simulink model "SigProcess"  (R2022b)
settings: Solver=FixedStepDiscrete  StartTime=0.0  StopTime=10.0  FixedStep=0.001  RelTol=1e-3
undefined symbols (not defined in the file): cClCddAdc_D_u16ADNum, cClCddAdc_D_u8FilterType, cClCddAdc_D_u8RawValueNum, cTmAfCtrl_Te_s32ShttrPosnColdOnHp
libraries: simulink x132
(part 2 of 7)

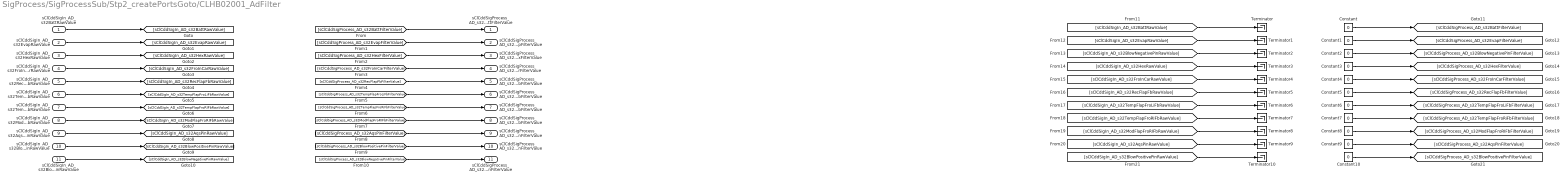
== system SigProcess/SigProcessSub/Stp2_createPortsGoto/CLHB02001_AdFilter ==
  sClCddSigIn_AD_s32BattRawValue : Inport  Description=低压电池AD值  OutDataTypeStr=single
  sClCddSigIn_AD_s32EvapRawValue : Inport  Description=空调箱蒸发器原始AD值  Port=2  OutDataTypeStr=single
  sClCddSigIn_AD_s32HexRawValue : Inport  Description=空调箱热交换器原始AD值  Port=3  OutDataTypeStr=single
  sClCddSigIn_AD_s32FroInCarRawValue : Inport  Description=前排车内温度传感器AD值  Port=4  OutDataTypeStr=single
  sClCddSigIn_AD_s32RecFlapFbRawValue : Inport  Description=内循环风门电机位置反馈  Port=5  OutDataTypeStr=single
  sClCddSigIn_AD_s32TempFlapFroLiFbRawValue : Inport  Description=前左风门电机位置反馈  Port=6  OutDataTypeStr=single
  sClCddSigIn_AD_s32TempFlapFroRIFbRawValue : Inport  Description=前右风门电机位置反馈  Port=7  OutMin=0  OutMax=2048  OutDataTypeStr=single
  sClCddSigIn_AD_s32ModFlapFroRIFbRawValue : Inport  Description=模式风门电机位置反馈  Port=8  OutMin=0  OutMax=2048  OutDataTypeStr=single
  sClCddSigIn_AD_s32AqsPinRawValue : Inport  Description=AQSPWM驱动芯片诊断PIN脚AD值  Port=9  OutMin=0  OutMax=2048  OutDataTypeStr=single
  sClCddSigIn_AD_s32BlowPositivePinRawValue : Inport  Description=鼓风机调速电机正极反馈  Port=10  OutMin=0  OutMax=2048  OutDataTypeStr=single
  sClCddSigIn_AD_s32BlowNegativePinRawValue : Inport  Description=鼓风机调速电机负极反馈  Port=11  OutMin=0  OutMax=2048  OutDataTypeStr=single
  Constant{,1..10} (11 alike) : Constant  Value=0  OutDataTypeStr=single
  Terminator{,1..10} (11 alike) : Terminator
  sClCddSigProcess_AD_s32BattFilterValue : Outport  Description=低压电池滤波后AD值  OutMin=0  OutMax=2048  OutDataTypeStr=single
  sClCddSigProcess_AD_s32EvapFilterValue : Outport  Description=空调箱蒸发器滤波后AD值  Port=2  OutMin=0  OutMax=2048  OutDataTypeStr=single
  sClCddSigProcess_AD_s32HexFilterValue : Outport  Description=空调箱热交换器滤波后AD值  Port=3  OutMin=0  OutMax=2048  OutDataTypeStr=single
  sClCddSigProcess_AD_s32FroInCarFilterValue : Outport  Description=前排车内温度传感器滤波后AD值  Port=4  OutMin=0  OutMax=2048  OutDataTypeStr=single
  sClCddSigProcess_AD_s32RecFlapFbFilterValue : Outport  Description=内循环风门电机位置反馈滤波值  Port=5  OutMin=0  OutMax=2048  OutDataTypeStr=single
  sClCddSigProcess_AD_s32TempFlapFroLiFbFilterValue : Outport  Description=前左风门电机位置反馈滤波值  Port=6  OutMin=0  OutMax=2048  OutDataTypeStr=single
  sClCddSigProcess_AD_s32TempFlapFroRiFbFilterValue : Outport  Description=前右风门电机位置反馈滤波值  Port=7  OutMin=0  OutMax=2048  OutDataTypeStr=single
  sClCddSigProcess_AD_s32ModFlapFroRIFbFilterValue : Outport  Description=模式风门电机位置反馈滤波值  Port=8  OutMin=0  OutMax=2048  OutDataTypeStr=single
  sClCddSigProcess_AD_s32AqsPinFilterValue : Outport  Description=AQSPWM驱动芯片诊断PIN脚滤波值  Port=9  OutMin=0  OutMax=2048  OutDataTypeStr=single
  sClCddSigProcess_AD_s32BlowPositivePinFilterValue : Outport  Description=鼓风机调速电机正极反馈滤波值  Port=10  OutMin=0  OutMax=2048  OutDataTypeStr=single
  sClCddSigProcess_AD_s32BlowNegativePinFilterValue : Outport  Description=鼓风机调速电机负极反馈滤波值  Port=11  OutMin=0  OutMax=2048  OutDataTypeStr=single
  wires:
  sClCddSigIn_AD_s32BattRawValue/1 -> [sClCddSigIn_AD_s32BattRawValue]
  sClCddSigIn_AD_s32EvapRawValue/1 -> [sClCddSigIn_AD_s32EvapRawValue]
  sClCddSigIn_AD_s32HexRawValue/1 -> [sClCddSigIn_AD_s32HexRawValue]
  sClCddSigIn_AD_s32FroInCarRawValue/1 -> [sClCddSigIn_AD_s32FroInCarRawValue]
  sClCddSigIn_AD_s32RecFlapFbRawValue/1 -> [sClCddSigIn_AD_s32RecFlapFbRawValue]
  sClCddSigIn_AD_s32TempFlapFroLiFbRawValue/1 -> [sClCddSigIn_AD_s32TempFlapFroLiFbRawValue]
  sClCddSigIn_AD_s32TempFlapFroRIFbRawValue/1 -> [sClCddSigIn_AD_s32TempFlapFroRIFbRawValue]
  sClCddSigIn_AD_s32ModFlapFroRIFbRawValue/1 -> [sClCddSigIn_AD_s32ModFlapFroRIFbRawValue]
  sClCddSigIn_AD_s32AqsPinRawValue/1 -> [sClCddSigIn_AD_s32AqsPinRawValue]
  sClCddSigIn_AD_s32BlowPositivePinRawValue/1 -> [sClCddSigIn_AD_s32BlowPositivePinRawValue]
  sClCddSigIn_AD_s32BlowNegativePinRawValue/1 -> [sClCddSigIn_AD_s32BlowNegativePinRawValue]
  [sClCddSigProcess_AD_s32BattFilterValue] -> sClCddSigProcess_AD_s32BattFilterValue/1
  [sClCddSigProcess_AD_s32EvapFilterValue] -> sClCddSigProcess_AD_s32EvapFilterValue/1
  [sClCddSigProcess_AD_s32HexFilterValue] -> sClCddSigProcess_AD_s32HexFilterValue/1
  [sClCddSigProcess_AD_s32FroInCarFilterValue] -> sClCddSigProcess_AD_s32FroInCarFilterValue/1
  [sClCddSigProcess_AD_s32RecFlapFbFilterValue] -> sClCddSigProcess_AD_s32RecFlapFbFilterValue/1
  [sClCddSigProcess_AD_s32TempFlapFroLiFbFilterValue] -> sClCddSigProcess_AD_s32TempFlapFroLiFbFilterValue/1
  [sClCddSigProcess_AD_s32TempFlapFroRiFbFilterValue] -> sClCddSigProcess_AD_s32TempFlapFroRiFbFilterValue/1
  [sClCddSigProcess_AD_s32ModFlapFroRIFbFilterValue] -> sClCddSigProcess_AD_s32ModFlapFroRIFbFilterValue/1
  [sClCddSigProcess_AD_s32AqsPinFilterValue] -> sClCddSigProcess_AD_s32AqsPinFilterValue/1
  [sClCddSigProcess_AD_s32BlowPositivePinFilterValue] -> sClCddSigProcess_AD_s32BlowPositivePinFilterValue/1
  [sClCddSigProcess_AD_s32BlowNegativePinFilterValue] -> sClCddSigProcess_AD_s32BlowNegativePinFilterValue/1
  Constant/1 -> [sClCddSigProcess_AD_s32BattFilterValue]
  Constant1/1 -> [sClCddSigProcess_AD_s32EvapFilterValue]
  Constant2/1 -> [sClCddSigProcess_AD_s32BlowNegativePinFilterValue]
  Constant3/1 -> [sClCddSigProcess_AD_s32HexFilterValue]
  Constant4/1 -> [sClCddSigProcess_AD_s32FroInCarFilterValue]
  Constant5/1 -> [sClCddSigProcess_AD_s32RecFlapFbFilterValue]
  Constant6/1 -> [sClCddSigProcess_AD_s32TempFlapFroLiFbFilterValue]
  Constant7/1 -> [sClCddSigProcess_AD_s32TempFlapFroRiFbFilterValue]
  Constant8/1 -> [sClCddSigProcess_AD_s32ModFlapFroRIFbFilterValue]
  Constant9/1 -> [sClCddSigProcess_AD_s32AqsPinFilterValue]
  Constant10/1 -> [sClCddSigProcess_AD_s32BlowPositivePinFilterValue]
  [sClCddSigIn_AD_s32BattRawValue] -> Terminator/1
  [sClCddSigIn_AD_s32EvapRawValue] -> Terminator1/1
  [sClCddSigIn_AD_s32BlowNegativePinRawValue] -> Terminator2/1
  [sClCddSigIn_AD_s32HexRawValue] -> Terminator3/1
  [sClCddSigIn_AD_s32FroInCarRawValue] -> Terminator4/1
  [sClCddSigIn_AD_s32RecFlapFbRawValue] -> Terminator5/1
  [sClCddSigIn_AD_s32TempFlapFroLiFbRawValue] -> Terminator6/1
  [sClCddSigIn_AD_s32TempFlapFroRIFbRawValue] -> Terminator7/1
  [sClCddSigIn_AD_s32ModFlapFroRIFbRawValue] -> Terminator8/1
  [sClCddSigIn_AD_s32AqsPinRawValue] -> Terminator9/1
  [sClCddSigIn_AD_s32BlowPositivePinRawValue] -> Terminator10/1

== system SigProcess/SigProcessSub/Stp2_createPortsGoto/CLHB02001_AdVoltChange ==

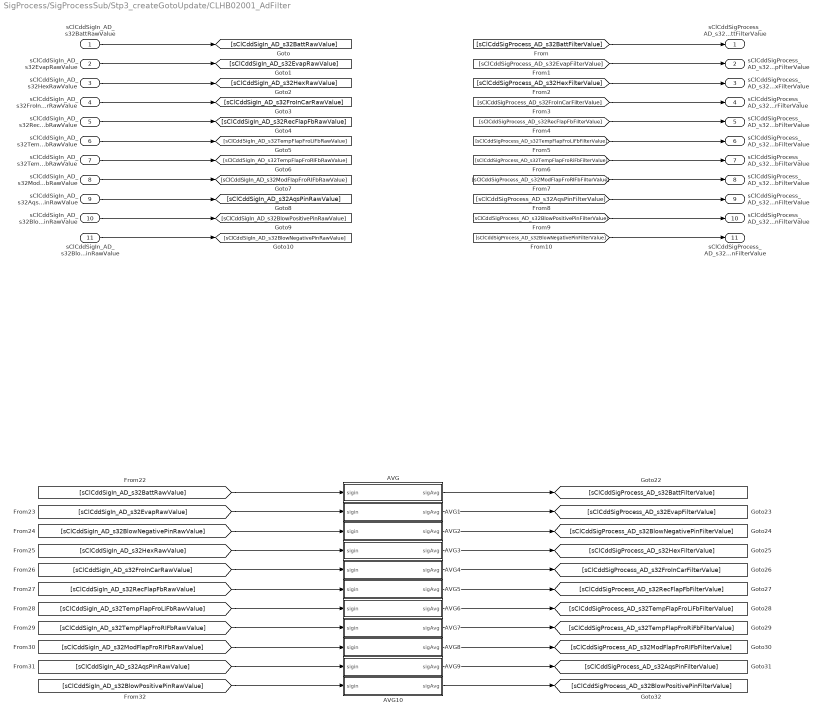
== system SigProcess/SigProcessSub/Stp3_createGotoUpdate/CLHB02001_AdFilter ==
  sClCddSigIn_AD_s32BattRawValue : Inport  Description=低压电池AD值  OutDataTypeStr=single
  sClCddSigIn_AD_s32EvapRawValue : Inport  Description=空调箱蒸发器原始AD值  Port=2  OutDataTypeStr=single
  sClCddSigIn_AD_s32HexRawValue : Inport  Description=空调箱热交换器原始AD值  Port=3  OutDataTypeStr=single
  sClCddSigIn_AD_s32FroInCarRawValue : Inport  Description=前排车内温度传感器AD值  Port=4  OutDataTypeStr=single
  sClCddSigIn_AD_s32RecFlapFbRawValue : Inport  Description=内循环风门电机位置反馈  Port=5  OutDataTypeStr=single
  sClCddSigIn_AD_s32TempFlapFroLiFbRawValue : Inport  Description=前左风门电机位置反馈  Port=6  OutDataTypeStr=single
  sClCddSigIn_AD_s32TempFlapFroRIFbRawValue : Inport  Description=前右风门电机位置反馈  Port=7  OutMin=0  OutMax=2048  OutDataTypeStr=single
  sClCddSigIn_AD_s32ModFlapFroRIFbRawValue : Inport  Description=模式风门电机位置反馈  Port=8  OutMin=0  OutMax=2048  OutDataTypeStr=single
  sClCddSigIn_AD_s32AqsPinRawValue : Inport  Description=AQSPWM驱动芯片诊断PIN脚AD值  Port=9  OutMin=0  OutMax=2048  OutDataTypeStr=single
  sClCddSigIn_AD_s32BlowPositivePinRawValue : Inport  Description=鼓风机调速电机正极反馈  Port=10  OutMin=0  OutMax=2048  OutDataTypeStr=single
  sClCddSigIn_AD_s32BlowNegativePinRawValue : Inport  Description=鼓风机调速电机负极反馈  Port=11  OutMin=0  OutMax=2048  OutDataTypeStr=single
  AVG : Subsystem
  AVG1 : Subsystem
  AVG10 : Subsystem
  AVG2 : Subsystem
  AVG3 : Subsystem
  AVG4 : Subsystem
  AVG5 : Subsystem
  AVG6 : Subsystem
  AVG7 : Subsystem
  AVG8 : Subsystem
  AVG9 : Subsystem
  sClCddSigProcess_AD_s32BattFilterValue : Outport  Description=低压电池滤波后AD值  OutMin=0  OutMax=2048  OutDataTypeStr=single
  sClCddSigProcess_AD_s32EvapFilterValue : Outport  Description=空调箱蒸发器滤波后AD值  Port=2  OutMin=0  OutMax=2048  OutDataTypeStr=single
  sClCddSigProcess_AD_s32HexFilterValue : Outport  Description=空调箱热交换器滤波后AD值  Port=3  OutMin=0  OutMax=2048  OutDataTypeStr=single
  sClCddSigProcess_AD_s32FroInCarFilterValue : Outport  Description=前排车内温度传感器滤波后AD值  Port=4  OutMin=0  OutMax=2048  OutDataTypeStr=single
  sClCddSigProcess_AD_s32RecFlapFbFilterValue : Outport  Description=内循环风门电机位置反馈滤波值  Port=5  OutMin=0  OutMax=2048  OutDataTypeStr=single
  sClCddSigProcess_AD_s32TempFlapFroLiFbFilterValue : Outport  Description=前左风门电机位置反馈滤波值  Port=6  OutMin=0  OutMax=2048  OutDataTypeStr=single
  sClCddSigProcess_AD_s32TempFlapFroRiFbFilterValue : Outport  Description=前右风门电机位置反馈滤波值  Port=7  OutMin=0  OutMax=2048  OutDataTypeStr=single
  sClCddSigProcess_AD_s32ModFlapFroRIFbFilterValue : Outport  Description=模式风门电机位置反馈滤波值  Port=8  OutMin=0  OutMax=2048  OutDataTypeStr=single
  sClCddSigProcess_AD_s32AqsPinFilterValue : Outport  Description=AQSPWM驱动芯片诊断PIN脚滤波值  Port=9  OutMin=0  OutMax=2048  OutDataTypeStr=single
  sClCddSigProcess_AD_s32BlowPositivePinFilterValue : Outport  Description=鼓风机调速电机正极反馈滤波值  Port=10  OutMin=0  OutMax=2048  OutDataTypeStr=single
  sClCddSigProcess_AD_s32BlowNegativePinFilterValue : Outport  Description=鼓风机调速电机负极反馈滤波值  Port=11  OutMin=0  OutMax=2048  OutDataTypeStr=single
  wires:
  [sClCddSigProcess_AD_s32BlowNegativePinFilterValue] -> sClCddSigProcess_AD_s32BlowNegativePinFilterValue/1
  [sClCddSigProcess_AD_s32BlowPositivePinFilterValue] -> sClCddSigProcess_AD_s32BlowPositivePinFilterValue/1
  [sClCddSigProcess_AD_s32AqsPinFilterValue] -> sClCddSigProcess_AD_s32AqsPinFilterValue/1
  [sClCddSigProcess_AD_s32ModFlapFroRIFbFilterValue] -> sClCddSigProcess_AD_s32ModFlapFroRIFbFilterValue/1
  [sClCddSigProcess_AD_s32TempFlapFroRiFbFilterValue] -> sClCddSigProcess_AD_s32TempFlapFroRiFbFilterValue/1
  [sClCddSigProcess_AD_s32TempFlapFroLiFbFilterValue] -> sClCddSigProcess_AD_s32TempFlapFroLiFbFilterValue/1
  [sClCddSigProcess_AD_s32RecFlapFbFilterValue] -> sClCddSigProcess_AD_s32RecFlapFbFilterValue/1
  [sClCddSigProcess_AD_s32FroInCarFilterValue] -> sClCddSigProcess_AD_s32FroInCarFilterValue/1
  [sClCddSigProcess_AD_s32HexFilterValue] -> sClCddSigProcess_AD_s32HexFilterValue/1
  [sClCddSigProcess_AD_s32EvapFilterValue] -> sClCddSigProcess_AD_s32EvapFilterValue/1
  [sClCddSigProcess_AD_s32BattFilterValue] -> sClCddSigProcess_AD_s32BattFilterValue/1
  sClCddSigIn_AD_s32BlowNegativePinRawValue/1 -> [sClCddSigIn_AD_s32BlowNegativePinRawValue]
  sClCddSigIn_AD_s32BlowPositivePinRawValue/1 -> [sClCddSigIn_AD_s32BlowPositivePinRawValue]
  sClCddSigIn_AD_s32AqsPinRawValue/1 -> [sClCddSigIn_AD_s32AqsPinRawValue]
  sClCddSigIn_AD_s32ModFlapFroRIFbRawValue/1 -> [sClCddSigIn_AD_s32ModFlapFroRIFbRawValue]
  sClCddSigIn_AD_s32TempFlapFroRIFbRawValue/1 -> [sClCddSigIn_AD_s32TempFlapFroRIFbRawValue]
  sClCddSigIn_AD_s32TempFlapFroLiFbRawValue/1 -> [sClCddSigIn_AD_s32TempFlapFroLiFbRawValue]
  sClCddSigIn_AD_s32RecFlapFbRawValue/1 -> [sClCddSigIn_AD_s32RecFlapFbRawValue]
  sClCddSigIn_AD_s32FroInCarRawValue/1 -> [sClCddSigIn_AD_s32FroInCarRawValue]
  sClCddSigIn_AD_s32HexRawValue/1 -> [sClCddSigIn_AD_s32HexRawValue]
  sClCddSigIn_AD_s32EvapRawValue/1 -> [sClCddSigIn_AD_s32EvapRawValue]
  sClCddSigIn_AD_s32BattRawValue/1 -> [sClCddSigIn_AD_s32BattRawValue]
  [sClCddSigIn_AD_s32RecFlapFbRawValue] -> AVG5/1(sigin)
  AVG8/1(sigAvg) -> [sClCddSigProcess_AD_s32ModFlapFroRIFbFilterValue]
  AVG10/1(sigAvg) -> [sClCddSigProcess_AD_s32BlowPositivePinFilterValue]
  [sClCddSigIn_AD_s32AqsPinRawValue] -> AVG9/1(sigin)
  AVG9/1(sigAvg) -> [sClCddSigProcess_AD_s32AqsPinFilterValue]
  AVG6/1(sigAvg) -> [sClCddSigProcess_AD_s32TempFlapFroLiFbFilterValue]
  [sClCddSigIn_AD_s32ModFlapFroRIFbRawValue] -> AVG8/1(sigin)
  [sClCddSigIn_AD_s32BlowNegativePinRawValue] -> AVG2/1(sigin)
  [sClCddSigIn_AD_s32EvapRawValue] -> AVG1/1(sigin)
  [sClCddSigIn_AD_s32BattRawValue] -> AVG/1(sigin)
  AVG/1(sigAvg) -> [sClCddSigProcess_AD_s32BattFilterValue]
  AVG1/1(sigAvg) -> [sClCddSigProcess_AD_s32EvapFilterValue]
  AVG5/1(sigAvg) -> [sClCddSigProcess_AD_s32RecFlapFbFilterValue]
  [sClCddSigIn_AD_s32FroInCarRawValue] -> AVG4/1(sigin)
  AVG4/1(sigAvg) -> [sClCddSigProcess_AD_s32FroInCarFilterValue]
  AVG2/1(sigAvg) -> [sClCddSigProcess_AD_s32BlowNegativePinFilterValue]
  [sClCddSigIn_AD_s32TempFlapFroRIFbRawValue] -> AVG7/1(sigin)
  [sClCddSigIn_AD_s32BlowPositivePinRawValue] -> AVG10/1(sigin)
  [sClCddSigIn_AD_s32HexRawValue] -> AVG3/1(sigin)
  AVG3/1(sigAvg) -> [sClCddSigProcess_AD_s32HexFilterValue]
  [sClCddSigIn_AD_s32TempFlapFroLiFbRawValue] -> AVG6/1(sigin)
  AVG7/1(sigAvg) -> [sClCddSigProcess_AD_s32TempFlapFroRiFbFilterValue]

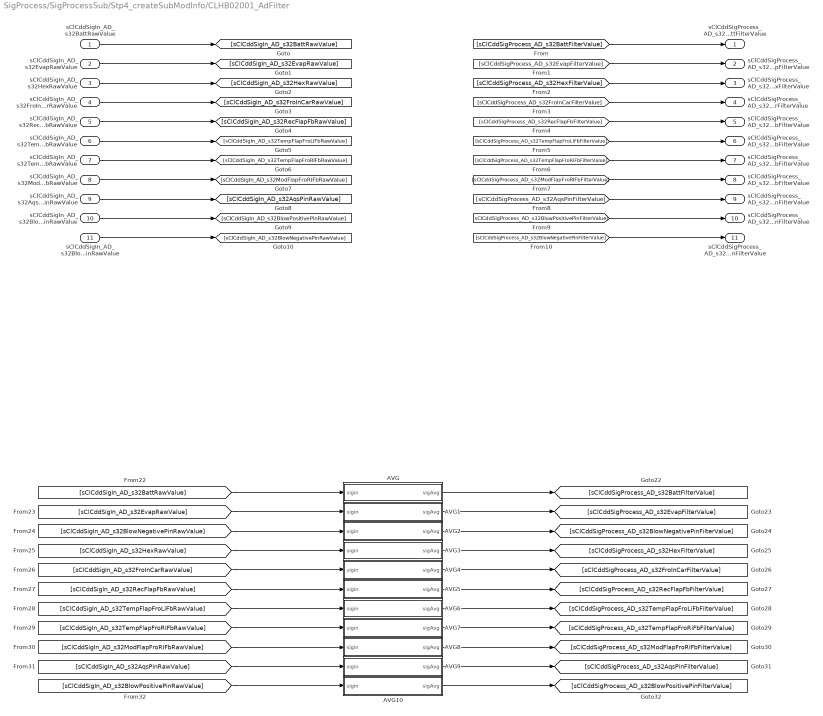
== system SigProcess/SigProcessSub/Stp4_createSubModInfo/CLHB02001_AdFilter ==
  sClCddSigIn_AD_s32BattRawValue : Inport  Description=低压电池AD值  OutDataTypeStr=single
  sClCddSigIn_AD_s32EvapRawValue : Inport  Description=空调箱蒸发器原始AD值  Port=2  OutDataTypeStr=single
  sClCddSigIn_AD_s32HexRawValue : Inport  Description=空调箱热交换器原始AD值  Port=3  OutDataTypeStr=single
  sClCddSigIn_AD_s32FroInCarRawValue : Inport  Description=前排车内温度传感器AD值  Port=4  OutDataTypeStr=single
  sClCddSigIn_AD_s32RecFlapFbRawValue : Inport  Description=内循环风门电机位置反馈  Port=5  OutDataTypeStr=single
  sClCddSigIn_AD_s32TempFlapFroLiFbRawValue : Inport  Description=前左风门电机位置反馈  Port=6  OutDataTypeStr=single
  sClCddSigIn_AD_s32TempFlapFroRIFbRawValue : Inport  Description=前右风门电机位置反馈  Port=7  OutMin=0  OutMax=2048  OutDataTypeStr=single
  sClCddSigIn_AD_s32ModFlapFroRIFbRawValue : Inport  Description=模式风门电机位置反馈  Port=8  OutMin=0  OutMax=2048  OutDataTypeStr=single
  sClCddSigIn_AD_s32AqsPinRawValue : Inport  Description=AQSPWM驱动芯片诊断PIN脚AD值  Port=9  OutMin=0  OutMax=2048  OutDataTypeStr=single
  sClCddSigIn_AD_s32BlowPositivePinRawValue : Inport  Description=鼓风机调速电机正极反馈  Port=10  OutMin=0  OutMax=2048  OutDataTypeStr=single
  sClCddSigIn_AD_s32BlowNegativePinRawValue : Inport  Description=鼓风机调速电机负极反馈  Port=11  OutMin=0  OutMax=2048  OutDataTypeStr=single
  AVG : Subsystem
  AVG1 : Subsystem
  AVG10 : Subsystem
  AVG2 : Subsystem
  AVG3 : Subsystem
  AVG4 : Subsystem
  AVG5 : Subsystem
  AVG6 : Subsystem
  AVG7 : Subsystem
  AVG8 : Subsystem
  AVG9 : Subsystem
  sClCddSigProcess_AD_s32BattFilterValue : Outport  Description=低压电池滤波后AD值  OutMin=0  OutMax=2048  OutDataTypeStr=single
  sClCddSigProcess_AD_s32EvapFilterValue : Outport  Description=空调箱蒸发器滤波后AD值  Port=2  OutMin=0  OutMax=2048  OutDataTypeStr=single
  sClCddSigProcess_AD_s32HexFilterValue : Outport  Description=空调箱热交换器滤波后AD值  Port=3  OutMin=0  OutMax=2048  OutDataTypeStr=single
  sClCddSigProcess_AD_s32FroInCarFilterValue : Outport  Description=前排车内温度传感器滤波后AD值  Port=4  OutMin=0  OutMax=2048  OutDataTypeStr=single
  sClCddSigProcess_AD_s32RecFlapFbFilterValue : Outport  Description=内循环风门电机位置反馈滤波值  Port=5  OutMin=0  OutMax=2048  OutDataTypeStr=single
  sClCddSigProcess_AD_s32TempFlapFroLiFbFilterValue : Outport  Description=前左风门电机位置反馈滤波值  Port=6  OutMin=0  OutMax=2048  OutDataTypeStr=single
  sClCddSigProcess_AD_s32TempFlapFroRiFbFilterValue : Outport  Description=前右风门电机位置反馈滤波值  Port=7  OutMin=0  OutMax=2048  OutDataTypeStr=single
  sClCddSigProcess_AD_s32ModFlapFroRIFbFilterValue : Outport  Description=模式风门电机位置反馈滤波值  Port=8  OutMin=0  OutMax=2048  OutDataTypeStr=single
  sClCddSigProcess_AD_s32AqsPinFilterValue : Outport  Description=AQSPWM驱动芯片诊断PIN脚滤波值  Port=9  OutMin=0  OutMax=2048  OutDataTypeStr=single
  sClCddSigProcess_AD_s32BlowPositivePinFilterValue : Outport  Description=鼓风机调速电机正极反馈滤波值  Port=10  OutMin=0  OutMax=2048  OutDataTypeStr=single
  sClCddSigProcess_AD_s32BlowNegativePinFilterValue : Outport  Description=鼓风机调速电机负极反馈滤波值  Port=11  OutMin=0  OutMax=2048  OutDataTypeStr=single
  wires:
  [sClCddSigProcess_AD_s32BlowNegativePinFilterValue] -> sClCddSigProcess_AD_s32BlowNegativePinFilterValue/1
  [sClCddSigProcess_AD_s32BlowPositivePinFilterValue] -> sClCddSigProcess_AD_s32BlowPositivePinFilterValue/1
  [sClCddSigProcess_AD_s32AqsPinFilterValue] -> sClCddSigProcess_AD_s32AqsPinFilterValue/1
  [sClCddSigProcess_AD_s32ModFlapFroRIFbFilterValue] -> sClCddSigProcess_AD_s32ModFlapFroRIFbFilterValue/1
  [sClCddSigProcess_AD_s32TempFlapFroRiFbFilterValue] -> sClCddSigProcess_AD_s32TempFlapFroRiFbFilterValue/1
  [sClCddSigProcess_AD_s32TempFlapFroLiFbFilterValue] -> sClCddSigProcess_AD_s32TempFlapFroLiFbFilterValue/1
  [sClCddSigProcess_AD_s32RecFlapFbFilterValue] -> sClCddSigProcess_AD_s32RecFlapFbFilterValue/1
  [sClCddSigProcess_AD_s32FroInCarFilterValue] -> sClCddSigProcess_AD_s32FroInCarFilterValue/1
  [sClCddSigProcess_AD_s32HexFilterValue] -> sClCddSigProcess_AD_s32HexFilterValue/1
  [sClCddSigProcess_AD_s32EvapFilterValue] -> sClCddSigProcess_AD_s32EvapFilterValue/1
  [sClCddSigProcess_AD_s32BattFilterValue] -> sClCddSigProcess_AD_s32BattFilterValue/1
  sClCddSigIn_AD_s32BlowNegativePinRawValue/1 -> [sClCddSigIn_AD_s32BlowNegativePinRawValue]
  sClCddSigIn_AD_s32BlowPositivePinRawValue/1 -> [sClCddSigIn_AD_s32BlowPositivePinRawValue]
  sClCddSigIn_AD_s32AqsPinRawValue/1 -> [sClCddSigIn_AD_s32AqsPinRawValue]
  sClCddSigIn_AD_s32ModFlapFroRIFbRawValue/1 -> [sClCddSigIn_AD_s32ModFlapFroRIFbRawValue]
  sClCddSigIn_AD_s32TempFlapFroRIFbRawValue/1 -> [sClCddSigIn_AD_s32TempFlapFroRIFbRawValue]
  sClCddSigIn_AD_s32TempFlapFroLiFbRawValue/1 -> [sClCddSigIn_AD_s32TempFlapFroLiFbRawValue]
  sClCddSigIn_AD_s32RecFlapFbRawValue/1 -> [sClCddSigIn_AD_s32RecFlapFbRawValue]
  sClCddSigIn_AD_s32FroInCarRawValue/1 -> [sClCddSigIn_AD_s32FroInCarRawValue]
  sClCddSigIn_AD_s32HexRawValue/1 -> [sClCddSigIn_AD_s32HexRawValue]
  sClCddSigIn_AD_s32EvapRawValue/1 -> [sClCddSigIn_AD_s32EvapRawValue]
  sClCddSigIn_AD_s32BattRawValue/1 -> [sClCddSigIn_AD_s32BattRawValue]
  [sClCddSigIn_AD_s32RecFlapFbRawValue] -> AVG5/1(sigin)
  AVG8/1(sigAvg) -> [sClCddSigProcess_AD_s32ModFlapFroRIFbFilterValue]
  AVG10/1(sigAvg) -> [sClCddSigProcess_AD_s32BlowPositivePinFilterValue]
  [sClCddSigIn_AD_s32AqsPinRawValue] -> AVG9/1(sigin)
  AVG9/1(sigAvg) -> [sClCddSigProcess_AD_s32AqsPinFilterValue]
  AVG6/1(sigAvg) -> [sClCddSigProcess_AD_s32TempFlapFroLiFbFilterValue]
  [sClCddSigIn_AD_s32ModFlapFroRIFbRawValue] -> AVG8/1(sigin)
  [sClCddSigIn_AD_s32BlowNegativePinRawValue] -> AVG2/1(sigin)
  [sClCddSigIn_AD_s32EvapRawValue] -> AVG1/1(sigin)
  [sClCddSigIn_AD_s32BattRawValue] -> AVG/1(sigin)
  AVG/1(sigAvg) -> [sClCddSigProcess_AD_s32BattFilterValue]
  AVG1/1(sigAvg) -> [sClCddSigProcess_AD_s32EvapFilterValue]
  AVG5/1(sigAvg) -> [sClCddSigProcess_AD_s32RecFlapFbFilterValue]
  [sClCddSigIn_AD_s32FroInCarRawValue] -> AVG4/1(sigin)
  AVG4/1(sigAvg) -> [sClCddSigProcess_AD_s32FroInCarFilterValue]
  AVG2/1(sigAvg) -> [sClCddSigProcess_AD_s32BlowNegativePinFilterValue]
  [sClCddSigIn_AD_s32TempFlapFroRIFbRawValue] -> AVG7/1(sigin)
  [sClCddSigIn_AD_s32BlowPositivePinRawValue] -> AVG10/1(sigin)
  [sClCddSigIn_AD_s32HexRawValue] -> AVG3/1(sigin)
  AVG3/1(sigAvg) -> [sClCddSigProcess_AD_s32HexFilterValue]
  [sClCddSigIn_AD_s32TempFlapFroLiFbRawValue] -> AVG6/1(sigin)
  AVG7/1(sigAvg) -> [sClCddSigProcess_AD_s32TempFlapFroRiFbFilterValue]

== system SigProcess/SigProcessSub/Stp5_ChangeAttrAndName/1_createPortGotoUpdate ==
  note: <模型信息: Stp4_createSubModInfo>
      |
      |
      | 【输入端口】
      | sClCddSigIn_AD_s32AqsPinRawValue
      | sClCddSigIn_AD_s32BattRawValue
      | sClCddSigIn_AD_s32BlowNegativePinRawValue
      | sClCddSigIn_AD_s32BlowPositivePinRawValue
      | sClCddSigIn_AD_s32EvapRawValue
      | sClCddSigIn_AD_s32FroInCarRawValue
      | sClCddSigIn_AD_s32HexRawValue
      | sClCddSigIn_AD_s32ModFlapFroRIFbRawValue
      | sClCddSigIn_AD_s32RecFlapFbRawValue
      | sClCddSigIn_AD_s32TempFlapFroLiFbRawValue
      | sClCddSigIn_AD_s32TempFlapFroRIFbRawValue
      |
      | 【输出端口】
      | sClCddSigProcess_AD_s32AqsPinFilterValue
      | sClCddSigProcess_AD_s32BattFilterValue
      | sClCddSigProcess_AD_s32BlowNegativePinFilterValue
      | sClCddSigProcess_AD_s32BlowPositivePinFilterValue
      | sClCddSigProcess_AD_s32EvapFilterValue
      | sClCddSigProcess_AD_s32FroInCarFilterValue
      | sClCddSigProcess_AD_s32HexFilterValue
      | sClCddSigProcess_AD_s32ModFlapFroRIFbFilterValue
      | sClCddSigProcess_AD_s32RecFlapFbFilterValue
      | sClCddSigProcess_AD_s32TempFlapFroLiFbFilterValue
      | sClCddSigProcess_AD_s32TempFlapFroRiFbFilterValue
      |
      | 【标定量】
      | 无标定量
      |
      | 创建时间: 2025-06-10 10:15:24
  sClCddSigIn_AD_s32AqsPinRawValue : Inport  OutDataTypeStr=single
  sClCddSigIn_AD_s32BattRawValue : Inport  Port=2  OutDataTypeStr=single
  sClCddSigIn_AD_s32BlowNegativePinRawValue : Inport  Port=3  OutDataTypeStr=single
  sClCddSigIn_AD_s32BlowPositivePinRawValue : Inport  Port=4  OutDataTypeStr=single
  sClCddSigIn_AD_s32EvapRawValue : Inport  Port=5  OutDataTypeStr=single
  sClCddSigIn_AD_s32FroInCarRawValue : Inport  Port=6  OutDataTypeStr=single
  sClCddSigIn_AD_s32HexRawValue : Inport  Port=7  OutDataTypeStr=single
  sClCddSigIn_AD_s32ModFlapFroRIFbRawValue : Inport  Port=8  OutDataTypeStr=single
  sClCddSigIn_AD_s32RecFlapFbRawValue : Inport  Port=9  OutDataTypeStr=single
  sClCddSigIn_AD_s32TempFlapFroLiFbRawValue : Inport  Port=10  OutDataTypeStr=single
  sClCddSigIn_AD_s32TempFlapFroRIFbRawValue : Inport  Port=11  OutDataTypeStr=single
  11_AdFilter : Subsystem
  sClCddSigProcess_AD_s32AqsPinFilterValue : Outport  OutDataTypeStr=single
  sClCddSigProcess_AD_s32BattFilterValue : Outport  Port=2  OutDataTypeStr=single
  sClCddSigProcess_AD_s32BlowNegativePinFilterValue : Outport  Port=3  OutDataTypeStr=single
  sClCddSigProcess_AD_s32BlowPositivePinFilterValue : Outport  Port=4  OutDataTypeStr=single
  sClCddSigProcess_AD_s32EvapFilterValue : Outport  Port=5  OutDataTypeStr=single
  sClCddSigProcess_AD_s32FroInCarFilterValue : Outport  Port=6  OutDataTypeStr=single
  sClCddSigProcess_AD_s32HexFilterValue : Outport  Port=7  OutDataTypeStr=single
  sClCddSigProcess_AD_s32ModFlapFroRIFbFilterValue : Outport  Port=8  OutDataTypeStr=single
  sClCddSigProcess_AD_s32RecFlapFbFilterValue : Outport  Port=9  OutDataTypeStr=single
  sClCddSigProcess_AD_s32TempFlapFroLiFbFilterValue : Outport  Port=10  OutDataTypeStr=single
  sClCddSigProcess_AD_s32TempFlapFroRiFbFilterValue : Outport  Port=11  OutDataTypeStr=single
  wires:
  [sClCddSigIn_AD_s32BattRawValue] -> 11_AdFilter/1(sClCddSigIn_AD_s32BattRawValue)
  [sClCddSigIn_AD_s32EvapRawValue] -> 11_AdFilter/2(sClCddSigIn_AD_s32EvapRawValue)
  [sClCddSigIn_AD_s32HexRawValue] -> 11_AdFilter/3(sClCddSigIn_AD_s32HexRawValue)
  [sClCddSigIn_AD_s32FroInCarRawValue] -> 11_AdFilter/4(sClCddSigIn_AD_s32FroInCarRawValue)
  [sClCddSigIn_AD_s32RecFlapFbRawValue] -> 11_AdFilter/5(sClCddSigIn_AD_s32RecFlapFbRawValue)
  [sClCddSigIn_AD_s32TempFlapFroLiFbRawValue] -> 11_AdFilter/6(sClCddSigIn_AD_s32TempFlapFroLiFbRawValue)
  [sClCddSigIn_AD_s32TempFlapFroRIFbRawValue] -> 11_AdFilter/7(sClCddSigIn_AD_s32TempFlapFroRIFbRawValue)
  [sClCddSigIn_AD_s32ModFlapFroRIFbRawValue] -> 11_AdFilter/8(sClCddSigIn_AD_s32ModFlapFroRIFbRawValue)
  [sClCddSigIn_AD_s32AqsPinRawValue] -> 11_AdFilter/9(sClCddSigIn_AD_s32AqsPinRawValue)
  [sClCddSigIn_AD_s32BlowPositivePinRawValue] -> 11_AdFilter/10(sClCddSigIn_AD_s32BlowPositivePinRawValue)
  [sClCddSigIn_AD_s32BlowNegativePinRawValue] -> 11_AdFilter/11(sClCddSigIn_AD_s32BlowNegativePinRawValue)
  11_AdFilter/1(sClCddSigProcess_AD_s32BattFilterValue) -> [sClCddSigProcess_AD_s32BattFilterValue]
  11_AdFilter/2(sClCddSigProcess_AD_s32EvapFilterValue) -> [sClCddSigProcess_AD_s32EvapFilterValue]
  11_AdFilter/3(sClCddSigProcess_AD_s32HexFilterValue) -> [sClCddSigProcess_AD_s32HexFilterValue]
  11_AdFilter/4(sClCddSigProcess_AD_s32FroInCarFilterValue) -> [sClCddSigProcess_AD_s32FroInCarFilterValue]
  11_AdFilter/5(sClCddSigProcess_AD_s32RecFlapFbFilterValue) -> [sClCddSigProcess_AD_s32RecFlapFbFilterValue]
  11_AdFilter/6(sClCddSigProcess_AD_s32TempFlapFroLiFbFilterValue) -> [sClCddSigProcess_AD_s32TempFlapFroLiFbFilterValue]
  11_AdFilter/7(sClCddSigProcess_AD_s32TempFlapFroRiFbFilterValue) -> [sClCddSigProcess_AD_s32TempFlapFroRiFbFilterValue]
  11_AdFilter/8(sClCddSigProcess_AD_s32ModFlapFroRIFbFilterValue) -> [sClCddSigProcess_AD_s32ModFlapFroRIFbFilterValue]
  11_AdFilter/9(sClCddSigProcess_AD_s32AqsPinFilterValue) -> [sClCddSigProcess_AD_s32AqsPinFilterValue]
  11_AdFilter/10(sClCddSigProcess_AD_s32BlowPositivePinFilterValue) -> [sClCddSigProcess_AD_s32BlowPositivePinFilterValue]
  11_AdFilter/11(sClCddSigProcess_AD_s32BlowNegativePinFilterValue) -> [sClCddSigProcess_AD_s32BlowNegativePinFilterValue]
  sClCddSigIn_AD_s32AqsPinRawValue/1 -> [sClCddSigIn_AD_s32AqsPinRawValue]
  sClCddSigIn_AD_s32BattRawValue/1 -> [sClCddSigIn_AD_s32BattRawValue]
  sClCddSigIn_AD_s32BlowNegativePinRawValue/1 -> [sClCddSigIn_AD_s32BlowNegativePinRawValue]
  sClCddSigIn_AD_s32BlowPositivePinRawValue/1 -> [sClCddSigIn_AD_s32BlowPositivePinRawValue]
  sClCddSigIn_AD_s32EvapRawValue/1 -> [sClCddSigIn_AD_s32EvapRawValue]
  sClCddSigIn_AD_s32FroInCarRawValue/1 -> [sClCddSigIn_AD_s32FroInCarRawValue]
  sClCddSigIn_AD_s32HexRawValue/1 -> [sClCddSigIn_AD_s32HexRawValue]
  sClCddSigIn_AD_s32ModFlapFroRIFbRawValue/1 -> [sClCddSigIn_AD_s32ModFlapFroRIFbRawValue]
  sClCddSigIn_AD_s32RecFlapFbRawValue/1 -> [sClCddSigIn_AD_s32RecFlapFbRawValue]
  sClCddSigIn_AD_s32TempFlapFroLiFbRawValue/1 -> [sClCddSigIn_AD_s32TempFlapFroLiFbRawValue]
  sClCddSigIn_AD_s32TempFlapFroRIFbRawValue/1 -> [sClCddSigIn_AD_s32TempFlapFroRIFbRawValue]
  [sClCddSigProcess_AD_s32AqsPinFilterValue] -> sClCddSigProcess_AD_s32AqsPinFilterValue/1
  [sClCddSigProcess_AD_s32BattFilterValue] -> sClCddSigProcess_AD_s32BattFilterValue/1
  [sClCddSigProcess_AD_s32BlowNegativePinFilterValue] -> sClCddSigProcess_AD_s32BlowNegativePinFilterValue/1
  [sClCddSigProcess_AD_s32BlowPositivePinFilterValue] -> sClCddSigProcess_AD_s32BlowPositivePinFilterValue/1
  [sClCddSigProcess_AD_s32EvapFilterValue] -> sClCddSigProcess_AD_s32EvapFilterValue/1
  [sClCddSigProcess_AD_s32FroInCarFilterValue] -> sClCddSigProcess_AD_s32FroInCarFilterValue/1
  [sClCddSigProcess_AD_s32HexFilterValue] -> sClCddSigProcess_AD_s32HexFilterValue/1
  [sClCddSigProcess_AD_s32ModFlapFroRIFbFilterValue] -> sClCddSigProcess_AD_s32ModFlapFroRIFbFilterValue/1
  [sClCddSigProcess_AD_s32RecFlapFbFilterValue] -> sClCddSigProcess_AD_s32RecFlapFbFilterValue/1
  [sClCddSigProcess_AD_s32TempFlapFroLiFbFilterValue] -> sClCddSigProcess_AD_s32TempFlapFroLiFbFilterValue/1
  [sClCddSigProcess_AD_s32TempFlapFroRiFbFilterValue] -> sClCddSigProcess_AD_s32TempFlapFroRiFbFilterValue/1

== system SigProcess/SigProcessSub/Stp5_ChangeAttrAndName/2_createPortGotoUpdate1 ==
  note: <模型信息: Stp4_createSubModInfo>
      |
      |
      | 【输入端口】
      | sClCddSigIn_AD_s32AqsPinRawValue
      | sClCddSigIn_AD_s32BattRawValue
      | sClCddSigIn_AD_s32BlowNegativePinRawValue
      | sClCddSigIn_AD_s32BlowPositivePinRawValue
      | sClCddSigIn_AD_s32EvapRawValue
      | sClCddSigIn_AD_s32FroInCarRawValue
      | sClCddSigIn_AD_s32HexRawValue
      | sClCddSigIn_AD_s32ModFlapFroRIFbRawValue
      | sClCddSigIn_AD_s32RecFlapFbRawValue
      | sClCddSigIn_AD_s32TempFlapFroLiFbRawValue
      | sClCddSigIn_AD_s32TempFlapFroRIFbRawValue
      |
      | 【输出端口】
      | sClCddSigProcess_AD_s32AqsPinFilterValue
      | sClCddSigProcess_AD_s32BattFilterValue
      | sClCddSigProcess_AD_s32BlowNegativePinFilterValue
      | sClCddSigProcess_AD_s32BlowPositivePinFilterValue
      | sClCddSigProcess_AD_s32EvapFilterValue
      | sClCddSigProcess_AD_s32FroInCarFilterValue
      | sClCddSigProcess_AD_s32HexFilterValue
      | sClCddSigProcess_AD_s32ModFlapFroRIFbFilterValue
      | sClCddSigProcess_AD_s32RecFlapFbFilterValue
      | sClCddSigProcess_AD_s32TempFlapFroLiFbFilterValue
      | sClCddSigProcess_AD_s32TempFlapFroRiFbFilterValue
      |
      | 【标定量】
      | 无标定量
      |
      | 创建时间: 2025-06-10 10:15:24
  sClCddSigIn_AD_s32AqsPinRawValue : Inport  OutDataTypeStr=single
  sClCddSigIn_AD_s32BattRawValue : Inport  Port=2  OutDataTypeStr=single
  sClCddSigIn_AD_s32BlowNegativePinRawValue : Inport  Port=3  OutDataTypeStr=single
  sClCddSigIn_AD_s32BlowPositivePinRawValue : Inport  Port=4  OutDataTypeStr=single
  sClCddSigIn_AD_s32EvapRawValue : Inport  Port=5  OutDataTypeStr=single
  sClCddSigIn_AD_s32FroInCarRawValue : Inport  Port=6  OutDataTypeStr=single
  sClCddSigIn_AD_s32HexRawValue : Inport  Port=7  OutDataTypeStr=single
  sClCddSigIn_AD_s32ModFlapFroRIFbRawValue : Inport  Port=8  OutDataTypeStr=single
  sClCddSigIn_AD_s32RecFlapFbRawValue : Inport  Port=9  OutDataTypeStr=single
  sClCddSigIn_AD_s32TempFlapFroLiFbRawValue : Inport  Port=10  OutDataTypeStr=single
  sClCddSigIn_AD_s32TempFlapFroRIFbRawValue : Inport  Port=11  OutDataTypeStr=single
  21_AdFilter : Subsystem
  sClCddSigProcess_AD_s32AqsPinFilterValue : Outport  OutDataTypeStr=single
  sClCddSigProcess_AD_s32BattFilterValue : Outport  Port=2  OutDataTypeStr=single
  sClCddSigProcess_AD_s32BlowNegativePinFilterValue : Outport  Port=3  OutDataTypeStr=single
  sClCddSigProcess_AD_s32BlowPositivePinFilterValue : Outport  Port=4  OutDataTypeStr=single
  sClCddSigProcess_AD_s32EvapFilterValue : Outport  Port=5  OutDataTypeStr=single
  sClCddSigProcess_AD_s32FroInCarFilterValue : Outport  Port=6  OutDataTypeStr=single
  sClCddSigProcess_AD_s32HexFilterValue : Outport  Port=7  OutDataTypeStr=single
  sClCddSigProcess_AD_s32ModFlapFroRIFbFilterValue : Outport  Port=8  OutDataTypeStr=single
  sClCddSigProcess_AD_s32RecFlapFbFilterValue : Outport  Port=9  OutDataTypeStr=single
  sClCddSigProcess_AD_s32TempFlapFroLiFbFilterValue : Outport  Port=10  OutDataTypeStr=single
  sClCddSigProcess_AD_s32TempFlapFroRiFbFilterValue : Outport  Port=11  OutDataTypeStr=single
  wires:
  [sClCddSigProcess_AD_s32TempFlapFroRiFbFilterValue] -> sClCddSigProcess_AD_s32TempFlapFroRiFbFilterValue/1
  [sClCddSigProcess_AD_s32TempFlapFroLiFbFilterValue] -> sClCddSigProcess_AD_s32TempFlapFroLiFbFilterValue/1
  [sClCddSigProcess_AD_s32RecFlapFbFilterValue] -> sClCddSigProcess_AD_s32RecFlapFbFilterValue/1
  [sClCddSigProcess_AD_s32ModFlapFroRIFbFilterValue] -> sClCddSigProcess_AD_s32ModFlapFroRIFbFilterValue/1
  [sClCddSigProcess_AD_s32HexFilterValue] -> sClCddSigProcess_AD_s32HexFilterValue/1
  [sClCddSigProcess_AD_s32FroInCarFilterValue] -> sClCddSigProcess_AD_s32FroInCarFilterValue/1
  [sClCddSigProcess_AD_s32EvapFilterValue] -> sClCddSigProcess_AD_s32EvapFilterValue/1
  [sClCddSigProcess_AD_s32BlowPositivePinFilterValue] -> sClCddSigProcess_AD_s32BlowPositivePinFilterValue/1
  [sClCddSigProcess_AD_s32BlowNegativePinFilterValue] -> sClCddSigProcess_AD_s32BlowNegativePinFilterValue/1
  [sClCddSigProcess_AD_s32BattFilterValue] -> sClCddSigProcess_AD_s32BattFilterValue/1
  [sClCddSigProcess_AD_s32AqsPinFilterValue] -> sClCddSigProcess_AD_s32AqsPinFilterValue/1
  sClCddSigIn_AD_s32TempFlapFroRIFbRawValue/1 -> [sClCddSigIn_AD_s32TempFlapFroRIFbRawValue]
  sClCddSigIn_AD_s32TempFlapFroLiFbRawValue/1 -> [sClCddSigIn_AD_s32TempFlapFroLiFbRawValue]
  sClCddSigIn_AD_s32RecFlapFbRawValue/1 -> [sClCddSigIn_AD_s32RecFlapFbRawValue]
  sClCddSigIn_AD_s32ModFlapFroRIFbRawValue/1 -> [sClCddSigIn_AD_s32ModFlapFroRIFbRawValue]
  sClCddSigIn_AD_s32HexRawValue/1 -> [sClCddSigIn_AD_s32HexRawValue]
  sClCddSigIn_AD_s32FroInCarRawValue/1 -> [sClCddSigIn_AD_s32FroInCarRawValue]
  sClCddSigIn_AD_s32EvapRawValue/1 -> [sClCddSigIn_AD_s32EvapRawValue]
  sClCddSigIn_AD_s32BlowPositivePinRawValue/1 -> [sClCddSigIn_AD_s32BlowPositivePinRawValue]
  sClCddSigIn_AD_s32BlowNegativePinRawValue/1 -> [sClCddSigIn_AD_s32BlowNegativePinRawValue]
  sClCddSigIn_AD_s32BattRawValue/1 -> [sClCddSigIn_AD_s32BattRawValue]
  sClCddSigIn_AD_s32AqsPinRawValue/1 -> [sClCddSigIn_AD_s32AqsPinRawValue]
  21_AdFilter/11(sClCddSigProcess_AD_s32BlowNegativePinFilterValue) -> [sClCddSigProcess_AD_s32BlowNegativePinFilterValue]
  21_AdFilter/10(sClCddSigProcess_AD_s32BlowPositivePinFilterValue) -> [sClCddSigProcess_AD_s32BlowPositivePinFilterValue]
  21_AdFilter/9(sClCddSigProcess_AD_s32AqsPinFilterValue) -> [sClCddSigProcess_AD_s32AqsPinFilterValue]
  21_AdFilter/8(sClCddSigProcess_AD_s32ModFlapFroRIFbFilterValue) -> [sClCddSigProcess_AD_s32ModFlapFroRIFbFilterValue]
  21_AdFilter/7(sClCddSigProcess_AD_s32TempFlapFroRiFbFilterValue) -> [sClCddSigProcess_AD_s32TempFlapFroRiFbFilterValue]
  21_AdFilter/6(sClCddSigProcess_AD_s32TempFlapFroLiFbFilterValue) -> [sClCddSigProcess_AD_s32TempFlapFroLiFbFilterValue]
  21_AdFilter/5(sClCddSigProcess_AD_s32RecFlapFbFilterValue) -> [sClCddSigProcess_AD_s32RecFlapFbFilterValue]
  21_AdFilter/4(sClCddSigProcess_AD_s32FroInCarFilterValue) -> [sClCddSigProcess_AD_s32FroInCarFilterValue]
  21_AdFilter/3(sClCddSigProcess_AD_s32HexFilterValue) -> [sClCddSigProcess_AD_s32HexFilterValue]
  21_AdFilter/2(sClCddSigProcess_AD_s32EvapFilterValue) -> [sClCddSigProcess_AD_s32EvapFilterValue]
  21_AdFilter/1(sClCddSigProcess_AD_s32BattFilterValue) -> [sClCddSigProcess_AD_s32BattFilterValue]
  [sClCddSigIn_AD_s32BlowNegativePinRawValue] -> 21_AdFilter/11(sClCddSigIn_AD_s32BlowNegativePinRawValue)
  [sClCddSigIn_AD_s32BlowPositivePinRawValue] -> 21_AdFilter/10(sClCddSigIn_AD_s32BlowPositivePinRawValue)
  [sClCddSigIn_AD_s32AqsPinRawValue] -> 21_AdFilter/9(sClCddSigIn_AD_s32AqsPinRawValue)
  [sClCddSigIn_AD_s32ModFlapFroRIFbRawValue] -> 21_AdFilter/8(sClCddSigIn_AD_s32ModFlapFroRIFbRawValue)
  [sClCddSigIn_AD_s32TempFlapFroRIFbRawValue] -> 21_AdFilter/7(sClCddSigIn_AD_s32TempFlapFroRIFbRawValue)
  [sClCddSigIn_AD_s32TempFlapFroLiFbRawValue] -> 21_AdFilter/6(sClCddSigIn_AD_s32TempFlapFroLiFbRawValue)
  [sClCddSigIn_AD_s32RecFlapFbRawValue] -> 21_AdFilter/5(sClCddSigIn_AD_s32RecFlapFbRawValue)
  [sClCddSigIn_AD_s32FroInCarRawValue] -> 21_AdFilter/4(sClCddSigIn_AD_s32FroInCarRawValue)
  [sClCddSigIn_AD_s32HexRawValue] -> 21_AdFilter/3(sClCddSigIn_AD_s32HexRawValue)
  [sClCddSigIn_AD_s32EvapRawValue] -> 21_AdFilter/2(sClCddSigIn_AD_s32EvapRawValue)
  [sClCddSigIn_AD_s32BattRawValue] -> 21_AdFilter/1(sClCddSigIn_AD_s32BattRawValue)

== system SigProcess/SigProcessSub/Stp5_ChangeAttrAndName/3_createPortGotoUpdate2 ==
  note: <模型信息: Stp4_createSubModInfo>
      |
      |
      | 【输入端口】
      | sClCddSigIn_AD_s32AqsPinRawValue
      | sClCddSigIn_AD_s32BattRawValue
      | sClCddSigIn_AD_s32BlowNegativePinRawValue
      | sClCddSigIn_AD_s32BlowPositivePinRawValue
      | sClCddSigIn_AD_s32EvapRawValue
      | sClCddSigIn_AD_s32FroInCarRawValue
      | sClCddSigIn_AD_s32HexRawValue
      | sClCddSigIn_AD_s32ModFlapFroRIFbRawValue
      | sClCddSigIn_AD_s32RecFlapFbRawValue
      | sClCddSigIn_AD_s32TempFlapFroLiFbRawValue
      | sClCddSigIn_AD_s32TempFlapFroRIFbRawValue
      |
      | 【输出端口】
      | sClCddSigProcess_AD_s32AqsPinFilterValue
      | sClCddSigProcess_AD_s32BattFilterValue
      | sClCddSigProcess_AD_s32BlowNegativePinFilterValue
      | sClCddSigProcess_AD_s32BlowPositivePinFilterValue
      | sClCddSigProcess_AD_s32EvapFilterValue
      | sClCddSigProcess_AD_s32FroInCarFilterValue
      | sClCddSigProcess_AD_s32HexFilterValue
      | sClCddSigProcess_AD_s32ModFlapFroRIFbFilterValue
      | sClCddSigProcess_AD_s32RecFlapFbFilterValue
      | sClCddSigProcess_AD_s32TempFlapFroLiFbFilterValue
      | sClCddSigProcess_AD_s32TempFlapFroRiFbFilterValue
      |
      | 【标定量】
      | 无标定量
      |
      | 创建时间: 2025-06-10 10:15:24
  sClCddSigIn_AD_s32AqsPinRawValue : Inport  OutDataTypeStr=single
  sClCddSigIn_AD_s32BattRawValue : Inport  Port=2  OutDataTypeStr=single
  sClCddSigIn_AD_s32BlowNegativePinRawValue : Inport  Port=3  OutDataTypeStr=single
  sClCddSigIn_AD_s32BlowPositivePinRawValue : Inport  Port=4  OutDataTypeStr=single
  sClCddSigIn_AD_s32EvapRawValue : Inport  Port=5  OutDataTypeStr=single
  sClCddSigIn_AD_s32FroInCarRawValue : Inport  Port=6  OutDataTypeStr=single
  sClCddSigIn_AD_s32HexRawValue : Inport  Port=7  OutDataTypeStr=single
  sClCddSigIn_AD_s32ModFlapFroRIFbRawValue : Inport  Port=8  OutDataTypeStr=single
  sClCddSigIn_AD_s32RecFlapFbRawValue : Inport  Port=9  OutDataTypeStr=single
  sClCddSigIn_AD_s32TempFlapFroLiFbRawValue : Inport  Port=10  OutDataTypeStr=single
  sClCddSigIn_AD_s32TempFlapFroRIFbRawValue : Inport  Port=11  OutDataTypeStr=single
  31_AdFilter : Subsystem
  sClCddSigProcess_AD_s32AqsPinFilterValue : Outport  OutDataTypeStr=single
  sClCddSigProcess_AD_s32BattFilterValue : Outport  Port=2  OutDataTypeStr=single
  sClCddSigProcess_AD_s32BlowNegativePinFilterValue : Outport  Port=3  OutDataTypeStr=single
  sClCddSigProcess_AD_s32BlowPositivePinFilterValue : Outport  Port=4  OutDataTypeStr=single
  sClCddSigProcess_AD_s32EvapFilterValue : Outport  Port=5  OutDataTypeStr=single
  sClCddSigProcess_AD_s32FroInCarFilterValue : Outport  Port=6  OutDataTypeStr=single
  sClCddSigProcess_AD_s32HexFilterValue : Outport  Port=7  OutDataTypeStr=single
  sClCddSigProcess_AD_s32ModFlapFroRIFbFilterValue : Outport  Port=8  OutDataTypeStr=single
  sClCddSigProcess_AD_s32RecFlapFbFilterValue : Outport  Port=9  OutDataTypeStr=single
  sClCddSigProcess_AD_s32TempFlapFroLiFbFilterValue : Outport  Port=10  OutDataTypeStr=single
  sClCddSigProcess_AD_s32TempFlapFroRiFbFilterValue : Outport  Port=11  OutDataTypeStr=single
  wires:
  [sClCddSigIn_AD_s32BattRawValue] -> 31_AdFilter/1(sClCddSigIn_AD_s32BattRawValue)
  [sClCddSigIn_AD_s32EvapRawValue] -> 31_AdFilter/2(sClCddSigIn_AD_s32EvapRawValue)
  [sClCddSigIn_AD_s32HexRawValue] -> 31_AdFilter/3(sClCddSigIn_AD_s32HexRawValue)
  [sClCddSigIn_AD_s32FroInCarRawValue] -> 31_AdFilter/4(sClCddSigIn_AD_s32FroInCarRawValue)
  [sClCddSigIn_AD_s32RecFlapFbRawValue] -> 31_AdFilter/5(sClCddSigIn_AD_s32RecFlapFbRawValue)
  [sClCddSigIn_AD_s32TempFlapFroLiFbRawValue] -> 31_AdFilter/6(sClCddSigIn_AD_s32TempFlapFroLiFbRawValue)
  [sClCddSigIn_AD_s32TempFlapFroRIFbRawValue] -> 31_AdFilter/7(sClCddSigIn_AD_s32TempFlapFroRIFbRawValue)
  [sClCddSigIn_AD_s32ModFlapFroRIFbRawValue] -> 31_AdFilter/8(sClCddSigIn_AD_s32ModFlapFroRIFbRawValue)
  [sClCddSigIn_AD_s32AqsPinRawValue] -> 31_AdFilter/9(sClCddSigIn_AD_s32AqsPinRawValue)
  [sClCddSigIn_AD_s32BlowPositivePinRawValue] -> 31_AdFilter/10(sClCddSigIn_AD_s32BlowPositivePinRawValue)
  [sClCddSigIn_AD_s32BlowNegativePinRawValue] -> 31_AdFilter/11(sClCddSigIn_AD_s32BlowNegativePinRawValue)
  31_AdFilter/1(sClCddSigProcess_AD_s32BattFilterValue) -> [sClCddSigProcess_AD_s32BattFilterValue]
  31_AdFilter/2(sClCddSigProcess_AD_s32EvapFilterValue) -> [sClCddSigProcess_AD_s32EvapFilterValue]
  31_AdFilter/3(sClCddSigProcess_AD_s32HexFilterValue) -> [sClCddSigProcess_AD_s32HexFilterValue]
  31_AdFilter/4(sClCddSigProcess_AD_s32FroInCarFilterValue) -> [sClCddSigProcess_AD_s32FroInCarFilterValue]
  31_AdFilter/5(sClCddSigProcess_AD_s32RecFlapFbFilterValue) -> [sClCddSigProcess_AD_s32RecFlapFbFilterValue]
  31_AdFilter/6(sClCddSigProcess_AD_s32TempFlapFroLiFbFilterValue) -> [sClCddSigProcess_AD_s32TempFlapFroLiFbFilterValue]
  31_AdFilter/7(sClCddSigProcess_AD_s32TempFlapFroRiFbFilterValue) -> [sClCddSigProcess_AD_s32TempFlapFroRiFbFilterValue]
  31_AdFilter/8(sClCddSigProcess_AD_s32ModFlapFroRIFbFilterValue) -> [sClCddSigProcess_AD_s32ModFlapFroRIFbFilterValue]
  31_AdFilter/9(sClCddSigProcess_AD_s32AqsPinFilterValue) -> [sClCddSigProcess_AD_s32AqsPinFilterValue]
  31_AdFilter/10(sClCddSigProcess_AD_s32BlowPositivePinFilterValue) -> [sClCddSigProcess_AD_s32BlowPositivePinFilterValue]
  31_AdFilter/11(sClCddSigProcess_AD_s32BlowNegativePinFilterValue) -> [sClCddSigProcess_AD_s32BlowNegativePinFilterValue]
  sClCddSigIn_AD_s32AqsPinRawValue/1 -> [sClCddSigIn_AD_s32AqsPinRawValue]
  sClCddSigIn_AD_s32BattRawValue/1 -> [sClCddSigIn_AD_s32BattRawValue]
  sClCddSigIn_AD_s32BlowNegativePinRawValue/1 -> [sClCddSigIn_AD_s32BlowNegativePinRawValue]
  sClCddSigIn_AD_s32BlowPositivePinRawValue/1 -> [sClCddSigIn_AD_s32BlowPositivePinRawValue]
  sClCddSigIn_AD_s32EvapRawValue/1 -> [sClCddSigIn_AD_s32EvapRawValue]
  sClCddSigIn_AD_s32FroInCarRawValue/1 -> [sClCddSigIn_AD_s32FroInCarRawValue]
  sClCddSigIn_AD_s32HexRawValue/1 -> [sClCddSigIn_AD_s32HexRawValue]
  sClCddSigIn_AD_s32ModFlapFroRIFbRawValue/1 -> [sClCddSigIn_AD_s32ModFlapFroRIFbRawValue]
  sClCddSigIn_AD_s32RecFlapFbRawValue/1 -> [sClCddSigIn_AD_s32RecFlapFbRawValue]
  sClCddSigIn_AD_s32TempFlapFroLiFbRawValue/1 -> [sClCddSigIn_AD_s32TempFlapFroLiFbRawValue]
  sClCddSigIn_AD_s32TempFlapFroRIFbRawValue/1 -> [sClCddSigIn_AD_s32TempFlapFroRIFbRawValue]
  [sClCddSigProcess_AD_s32AqsPinFilterValue] -> sClCddSigProcess_AD_s32AqsPinFilterValue/1
  [sClCddSigProcess_AD_s32BattFilterValue] -> sClCddSigProcess_AD_s32BattFilterValue/1
  [sClCddSigProcess_AD_s32BlowNegativePinFilterValue] -> sClCddSigProcess_AD_s32BlowNegativePinFilterValue/1
  [sClCddSigProcess_AD_s32BlowPositivePinFilterValue] -> sClCddSigProcess_AD_s32BlowPositivePinFilterValue/1
  [sClCddSigProcess_AD_s32EvapFilterValue] -> sClCddSigProcess_AD_s32EvapFilterValue/1
  [sClCddSigProcess_AD_s32FroInCarFilterValue] -> sClCddSigProcess_AD_s32FroInCarFilterValue/1
  [sClCddSigProcess_AD_s32HexFilterValue] -> sClCddSigProcess_AD_s32HexFilterValue/1
  [sClCddSigProcess_AD_s32ModFlapFroRIFbFilterValue] -> sClCddSigProcess_AD_s32ModFlapFroRIFbFilterValue/1
  [sClCddSigProcess_AD_s32RecFlapFbFilterValue] -> sClCddSigProcess_AD_s32RecFlapFbFilterValue/1
  [sClCddSigProcess_AD_s32TempFlapFroLiFbFilterValue] -> sClCddSigProcess_AD_s32TempFlapFroLiFbFilterValue/1
  [sClCddSigProcess_AD_s32TempFlapFroRiFbFilterValue] -> sClCddSigProcess_AD_s32TempFlapFroRiFbFilterValue/1

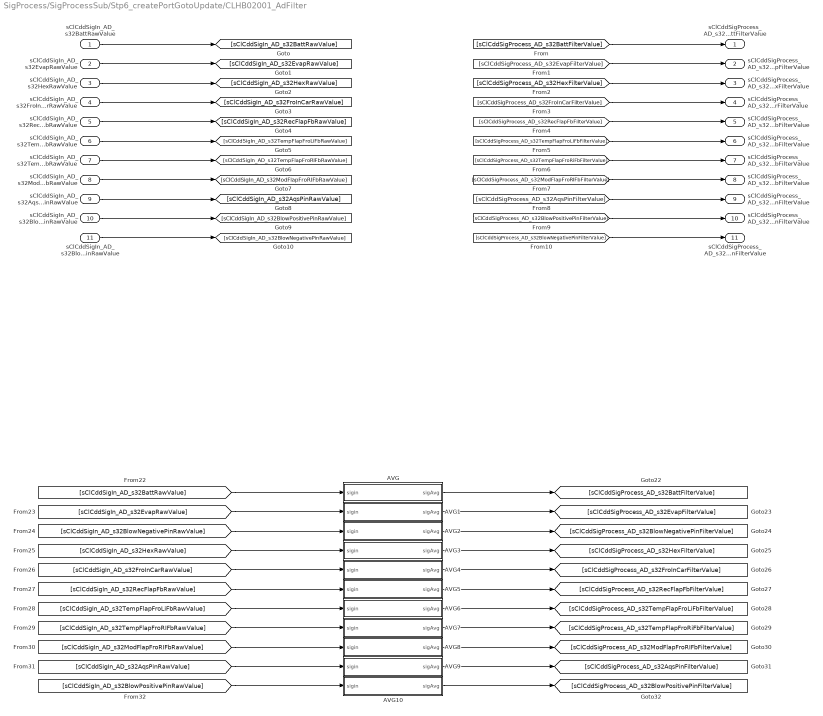
== system SigProcess/SigProcessSub/Stp6_createPortGotoUpdate/CLHB02001_AdFilter ==
  sClCddSigIn_AD_s32BattRawValue : Inport  Description=低压电池AD值  OutDataTypeStr=single
  sClCddSigIn_AD_s32EvapRawValue : Inport  Description=空调箱蒸发器原始AD值  Port=2  OutDataTypeStr=single
  sClCddSigIn_AD_s32HexRawValue : Inport  Description=空调箱热交换器原始AD值  Port=3  OutDataTypeStr=single
  sClCddSigIn_AD_s32FroInCarRawValue : Inport  Description=前排车内温度传感器AD值  Port=4  OutDataTypeStr=single
  sClCddSigIn_AD_s32RecFlapFbRawValue : Inport  Description=内循环风门电机位置反馈  Port=5  OutDataTypeStr=single
  sClCddSigIn_AD_s32TempFlapFroLiFbRawValue : Inport  Description=前左风门电机位置反馈  Port=6  OutDataTypeStr=single
  sClCddSigIn_AD_s32TempFlapFroRIFbRawValue : Inport  Description=前右风门电机位置反馈  Port=7  OutMin=0  OutMax=2048  OutDataTypeStr=single
  sClCddSigIn_AD_s32ModFlapFroRIFbRawValue : Inport  Description=模式风门电机位置反馈  Port=8  OutMin=0  OutMax=2048  OutDataTypeStr=single
  sClCddSigIn_AD_s32AqsPinRawValue : Inport  Description=AQSPWM驱动芯片诊断PIN脚AD值  Port=9  OutMin=0  OutMax=2048  OutDataTypeStr=single
  sClCddSigIn_AD_s32BlowPositivePinRawValue : Inport  Description=鼓风机调速电机正极反馈  Port=10  OutMin=0  OutMax=2048  OutDataTypeStr=single
  sClCddSigIn_AD_s32BlowNegativePinRawValue : Inport  Description=鼓风机调速电机负极反馈  Port=11  OutMin=0  OutMax=2048  OutDataTypeStr=single
  AVG : Subsystem
  AVG1 : Subsystem
  AVG10 : Subsystem
  AVG2 : Subsystem
  AVG3 : Subsystem
  AVG4 : Subsystem
  AVG5 : Subsystem
  AVG6 : Subsystem
  AVG7 : Subsystem
  AVG8 : Subsystem
  AVG9 : Subsystem
  sClCddSigProcess_AD_s32BattFilterValue : Outport  Description=低压电池滤波后AD值  OutMin=0  OutMax=2048  OutDataTypeStr=single
  sClCddSigProcess_AD_s32EvapFilterValue : Outport  Description=空调箱蒸发器滤波后AD值  Port=2  OutMin=0  OutMax=2048  OutDataTypeStr=single
  sClCddSigProcess_AD_s32HexFilterValue : Outport  Description=空调箱热交换器滤波后AD值  Port=3  OutMin=0  OutMax=2048  OutDataTypeStr=single
  sClCddSigProcess_AD_s32FroInCarFilterValue : Outport  Description=前排车内温度传感器滤波后AD值  Port=4  OutMin=0  OutMax=2048  OutDataTypeStr=single
  sClCddSigProcess_AD_s32RecFlapFbFilterValue : Outport  Description=内循环风门电机位置反馈滤波值  Port=5  OutMin=0  OutMax=2048  OutDataTypeStr=single
  sClCddSigProcess_AD_s32TempFlapFroLiFbFilterValue : Outport  Description=前左风门电机位置反馈滤波值  Port=6  OutMin=0  OutMax=2048  OutDataTypeStr=single
  sClCddSigProcess_AD_s32TempFlapFroRiFbFilterValue : Outport  Description=前右风门电机位置反馈滤波值  Port=7  OutMin=0  OutMax=2048  OutDataTypeStr=single
  sClCddSigProcess_AD_s32ModFlapFroRIFbFilterValue : Outport  Description=模式风门电机位置反馈滤波值  Port=8  OutMin=0  OutMax=2048  OutDataTypeStr=single
  sClCddSigProcess_AD_s32AqsPinFilterValue : Outport  Description=AQSPWM驱动芯片诊断PIN脚滤波值  Port=9  OutMin=0  OutMax=2048  OutDataTypeStr=single
  sClCddSigProcess_AD_s32BlowPositivePinFilterValue : Outport  Description=鼓风机调速电机正极反馈滤波值  Port=10  OutMin=0  OutMax=2048  OutDataTypeStr=single
  sClCddSigProcess_AD_s32BlowNegativePinFilterValue : Outport  Description=鼓风机调速电机负极反馈滤波值  Port=11  OutMin=0  OutMax=2048  OutDataTypeStr=single
  wires:
  [sClCddSigProcess_AD_s32BlowNegativePinFilterValue] -> sClCddSigProcess_AD_s32BlowNegativePinFilterValue/1
  [sClCddSigProcess_AD_s32BlowPositivePinFilterValue] -> sClCddSigProcess_AD_s32BlowPositivePinFilterValue/1
  [sClCddSigProcess_AD_s32AqsPinFilterValue] -> sClCddSigProcess_AD_s32AqsPinFilterValue/1
  [sClCddSigProcess_AD_s32ModFlapFroRIFbFilterValue] -> sClCddSigProcess_AD_s32ModFlapFroRIFbFilterValue/1
  [sClCddSigProcess_AD_s32TempFlapFroRiFbFilterValue] -> sClCddSigProcess_AD_s32TempFlapFroRiFbFilterValue/1
  [sClCddSigProcess_AD_s32TempFlapFroLiFbFilterValue] -> sClCddSigProcess_AD_s32TempFlapFroLiFbFilterValue/1
  [sClCddSigProcess_AD_s32RecFlapFbFilterValue] -> sClCddSigProcess_AD_s32RecFlapFbFilterValue/1
  [sClCddSigProcess_AD_s32FroInCarFilterValue] -> sClCddSigProcess_AD_s32FroInCarFilterValue/1
  [sClCddSigProcess_AD_s32HexFilterValue] -> sClCddSigProcess_AD_s32HexFilterValue/1
  [sClCddSigProcess_AD_s32EvapFilterValue] -> sClCddSigProcess_AD_s32EvapFilterValue/1
  [sClCddSigProcess_AD_s32BattFilterValue] -> sClCddSigProcess_AD_s32BattFilterValue/1
  sClCddSigIn_AD_s32BlowNegativePinRawValue/1 -> [sClCddSigIn_AD_s32BlowNegativePinRawValue]
  sClCddSigIn_AD_s32BlowPositivePinRawValue/1 -> [sClCddSigIn_AD_s32BlowPositivePinRawValue]
  sClCddSigIn_AD_s32AqsPinRawValue/1 -> [sClCddSigIn_AD_s32AqsPinRawValue]
  sClCddSigIn_AD_s32ModFlapFroRIFbRawValue/1 -> [sClCddSigIn_AD_s32ModFlapFroRIFbRawValue]
  sClCddSigIn_AD_s32TempFlapFroRIFbRawValue/1 -> [sClCddSigIn_AD_s32TempFlapFroRIFbRawValue]
  sClCddSigIn_AD_s32TempFlapFroLiFbRawValue/1 -> [sClCddSigIn_AD_s32TempFlapFroLiFbRawValue]
  sClCddSigIn_AD_s32RecFlapFbRawValue/1 -> [sClCddSigIn_AD_s32RecFlapFbRawValue]
  sClCddSigIn_AD_s32FroInCarRawValue/1 -> [sClCddSigIn_AD_s32FroInCarRawValue]
  sClCddSigIn_AD_s32HexRawValue/1 -> [sClCddSigIn_AD_s32HexRawValue]
  sClCddSigIn_AD_s32EvapRawValue/1 -> [sClCddSigIn_AD_s32EvapRawValue]
  sClCddSigIn_AD_s32BattRawValue/1 -> [sClCddSigIn_AD_s32BattRawValue]
  [sClCddSigIn_AD_s32RecFlapFbRawValue] -> AVG5/1(sigin)
  AVG8/1(sigAvg) -> [sClCddSigProcess_AD_s32ModFlapFroRIFbFilterValue]
  AVG10/1(sigAvg) -> [sClCddSigProcess_AD_s32BlowPositivePinFilterValue]
  [sClCddSigIn_AD_s32AqsPinRawValue] -> AVG9/1(sigin)
  AVG9/1(sigAvg) -> [sClCddSigProcess_AD_s32AqsPinFilterValue]
  AVG6/1(sigAvg) -> [sClCddSigProcess_AD_s32TempFlapFroLiFbFilterValue]
  [sClCddSigIn_AD_s32ModFlapFroRIFbRawValue] -> AVG8/1(sigin)
  [sClCddSigIn_AD_s32BlowNegativePinRawValue] -> AVG2/1(sigin)
  [sClCddSigIn_AD_s32EvapRawValue] -> AVG1/1(sigin)
  [sClCddSigIn_AD_s32BattRawValue] -> AVG/1(sigin)
  AVG/1(sigAvg) -> [sClCddSigProcess_AD_s32BattFilterValue]
  AVG1/1(sigAvg) -> [sClCddSigProcess_AD_s32EvapFilterValue]
  AVG5/1(sigAvg) -> [sClCddSigProcess_AD_s32RecFlapFbFilterValue]
  [sClCddSigIn_AD_s32FroInCarRawValue] -> AVG4/1(sigin)
  AVG4/1(sigAvg) -> [sClCddSigProcess_AD_s32FroInCarFilterValue]
  AVG2/1(sigAvg) -> [sClCddSigProcess_AD_s32BlowNegativePinFilterValue]
  [sClCddSigIn_AD_s32TempFlapFroRIFbRawValue] -> AVG7/1(sigin)
  [sClCddSigIn_AD_s32BlowPositivePinRawValue] -> AVG10/1(sigin)
  [sClCddSigIn_AD_s32HexRawValue] -> AVG3/1(sigin)
  AVG3/1(sigAvg) -> [sClCddSigProcess_AD_s32HexFilterValue]
  [sClCddSigIn_AD_s32TempFlapFroLiFbRawValue] -> AVG6/1(sigin)
  AVG7/1(sigAvg) -> [sClCddSigProcess_AD_s32TempFlapFroRiFbFilterValue]
